simulink model "third"  (R2024a)
settings: Solver=FixedStepAuto  StartTime=0.0  StopTime=15  FixedStep=0.00001  RelTol=1e-3
values from neighbouring files (symbols this model uses):
  Am1 = [cos(T1*omega1) sin(T1*omega1); -sin(T1*omega1) cos(T1*omega1)]    [third_calc1.m]
  ksi1 = [ksi10_1; ksi20_1]    [third_calc1.m]
  T = 0.2    [first_calc.m]
  T1 = 0.2    [third_calc1.m]
undefined symbols (not defined in the file or in its folder): Am, ksi, ksi10, ksi20, ksi30
settings Model: Creator=ventus  LastModifiedBy=ventus

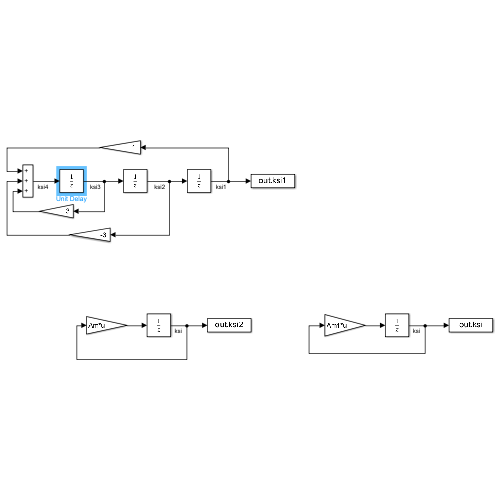
[thumbnail: Simulink's stored preview of the top-level diagram]
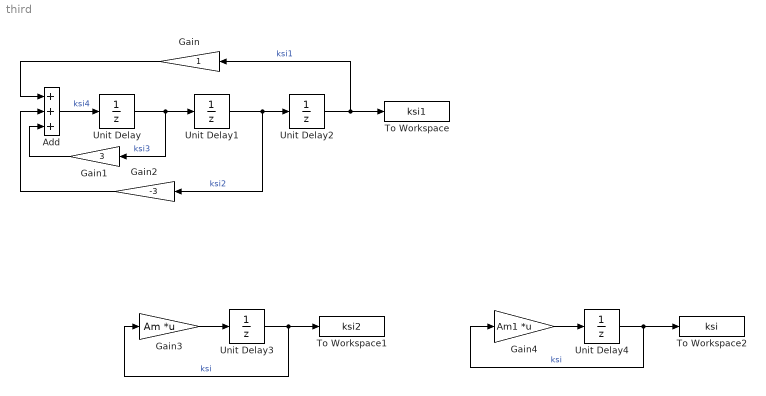
== system third ==
  Add : Sum  Inputs=+++
  Gain : Gain
  Gain1 : Gain  Gain=3
  Gain2 : Gain  Gain=-3
  Gain3 : Gain  Gain=Am  Multiplication=Matrix(K*u)
  Gain4 : Gain  Gain=Am1  Multiplication=Matrix(K*u)
  To Workspace : ToWorkspace  VariableName=ksi1  SaveFormat=Timeseries  SampleTime=-1
  To Workspace1 : ToWorkspace  VariableName=ksi2  SaveFormat=Timeseries  SampleTime=-1
  To Workspace2 : ToWorkspace  VariableName=ksi  SaveFormat=Timeseries  SampleTime=-1
  Unit Delay : UnitDelay  InitialCondition=ksi30  SampleTime=T  HasFrameUpgradeWarning=on
  Unit Delay1 : UnitDelay  InitialCondition=ksi20  SampleTime=T  HasFrameUpgradeWarning=on
  Unit Delay2 : UnitDelay  InitialCondition=ksi10  SampleTime=T  HasFrameUpgradeWarning=on
  Unit Delay3 : UnitDelay  InitialCondition=ksi  SampleTime=T  HasFrameUpgradeWarning=on
  Unit Delay4 : UnitDelay  InitialCondition=ksi1  SampleTime=T1  HasFrameUpgradeWarning=on
  wires:
  Unit Delay/1 -> Unit Delay1/1, Gain1/1  "ksi3"
  Unit Delay1/1 -> Unit Delay2/1, Gain2/1  "ksi2"
  Unit Delay2/1 -> Gain/1, To Workspace/1  "ksi1"
  Add/1 -> Unit Delay/1  "ksi4"
  Gain/1 -> Add/1
  Gain1/1 -> Add/3
  Gain2/1 -> Add/2
  Gain3/1 -> Unit Delay3/1
  Unit Delay3/1 -> To Workspace1/1, Gain3/1  "ksi"
  Unit Delay4/1 -> To Workspace2/1, Gain4/1  "ksi"
  Gain4/1 -> Unit Delay4/1
